simulink model "Retroacao_de_estados_3a_Lei_simulink"  (R2019a)
settings: Solver=VariableStepAuto  StartTime=0.0  StopTime=2  RelTol=1e-3
values from neighbouring files (symbols this model uses):
  a = [-1 1; 1 -2]    [Ganhos_observador_de_estados.m]    (also in Observador_de_estados.m; Retroacao_de_estados_1a_Lei.m = [0 1; -40 -3]; Retroacao_de_estados_2a_Lei.m = [[0 1]; [0 -50]])
  b = [1;0]    [Ganhos_observador_de_estados.m]    (also in Observador_de_estados.m; Retroacao_de_estados_1a_Lei.m = [0 ; 40]; Retroacao_de_estados_2a_Lei.m = [0;1370])
  c = [1 0]    [Ganhos_observador_de_estados.m]    (also in Observador_de_estados.m; Retroacao_de_estados_2a_Lei.m = eye(2))
  d = 0    [Retroacao_de_estados_2a_Lei.m]
  K1 = K(1)    [Retroacao_de_estados_1a_Lei.m]    (also in Retroacao_de_estados_2a_Lei.m; Retroacao_de_estados_3a_Lei.m)
  KI = -K(2)    [Retroacao_de_estados_3a_Lei.m]
settings Model: Creator=mathe  LastModifiedBy=vinic

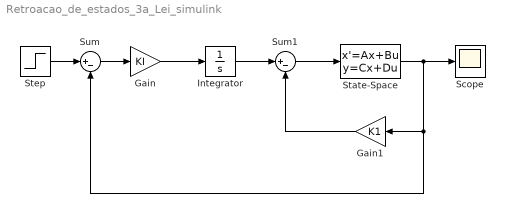
== system Retroacao_de_estados_3a_Lei_simulink ==
  Gain : Gain  Gain=KI
  Gain1 : Gain  Gain=K1
  Integrator : Integrator
  Scope : Scope
  State-Space : StateSpace  A=a  B=b  C=c  D=d  InitialCondition=0
  Step : Step  Time=0  SampleTime=0
  Sum : Sum  Inputs=|+-
  Sum1 : Sum  Inputs=|+-
  wires:
  Step/1 -> Sum/1
  Sum/1 -> Gain/1
  Gain/1 -> Integrator/1
  Integrator/1 -> Sum1/1
  Sum1/1 -> State-Space/1
  Gain1/1 -> Sum1/2
  State-Space/1 -> Sum/2, Gain1/1, Scope/1
